simulink model "TST_CoME_ShutOff"  (R2016b)
settings: Solver=FixedStepDiscrete  StartTime=0.0  StopTime=simTime  FixedStep=sampleTime  RelTol=1e-3
values from neighbouring files (symbols this model uses):
  testCase = 1    [initTST_CoME_ShutOff_001.m]    (also in initTST_CoME_ShutOff_002.m = 2; initTST_CoME_ShutOff_003.m = 3; initTST_CoME_ShutOff_004.m = 4)
libraries: simulink x17, UnitTest_Lib x12
settings Model: Creator=zhengjinyan  LastModifiedBy=zhengjinyan
settings DebuggingCC: SignalRangeChecking=error

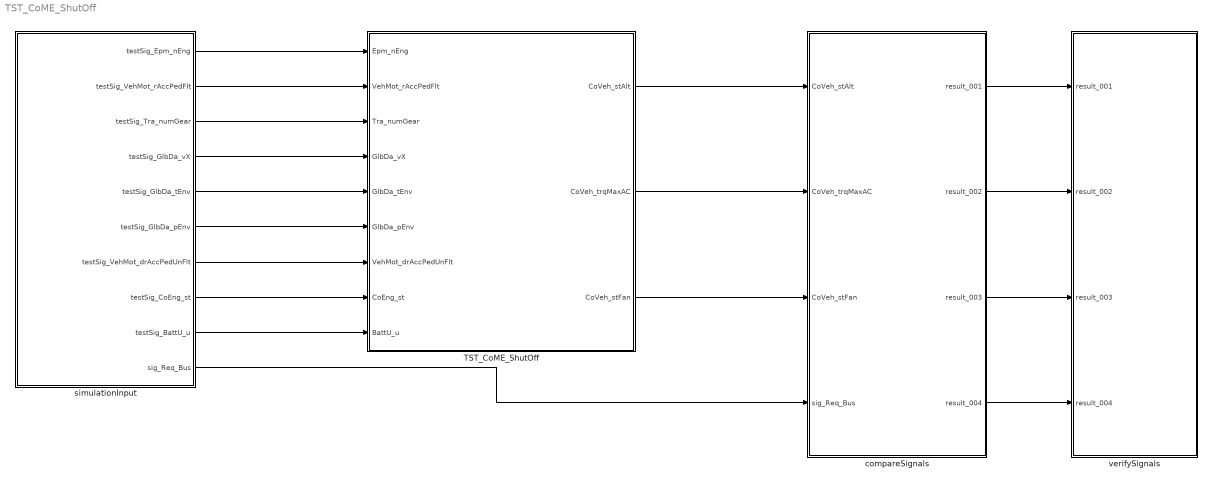
== system TST_CoME_ShutOff ==
  TST_CoME_ShutOff : Subsystem
  compareSignals : Subsystem
  simulationInput : Subsystem
  verifySignals : Subsystem
  wires:
  simulationInput/1(testSig_Epm_nEng) -> TST_CoME_ShutOff/1(Epm_nEng)
  simulationInput/2(testSig_VehMot_rAccPedFlt) -> TST_CoME_ShutOff/2(VehMot_rAccPedFlt)
  simulationInput/3(testSig_Tra_numGear) -> TST_CoME_ShutOff/3(Tra_numGear)
  simulationInput/4(testSig_GlbDa_vX) -> TST_CoME_ShutOff/4(GlbDa_vX)
  simulationInput/5(testSig_GlbDa_tEnv) -> TST_CoME_ShutOff/5(GlbDa_tEnv)
  simulationInput/6(testSig_GlbDa_pEnv) -> TST_CoME_ShutOff/6(GlbDa_pEnv)
  simulationInput/7(testSig_VehMot_drAccPedUnFlt) -> TST_CoME_ShutOff/7(VehMot_drAccPedUnFlt)
  simulationInput/8(testSig_CoEng_st) -> TST_CoME_ShutOff/8(CoEng_st)
  simulationInput/9(testSig_BattU_u) -> TST_CoME_ShutOff/9(BattU_u)
  TST_CoME_ShutOff/1(CoVeh_stAlt) -> compareSignals/1(CoVeh_stAlt)
  TST_CoME_ShutOff/2(CoVeh_trqMaxAC) -> compareSignals/2(CoVeh_trqMaxAC)
  TST_CoME_ShutOff/3(CoVeh_stFan) -> compareSignals/3(CoVeh_stFan)
  simulationInput/10(sig_Req_Bus) -> compareSignals/4(sig_Req_Bus)
  compareSignals/1(result_001) -> verifySignals/1(result_001)
  compareSignals/2(result_002) -> verifySignals/2(result_002)
  compareSignals/3(result_003) -> verifySignals/3(result_003)
  compareSignals/4(result_004) -> verifySignals/4(result_004)

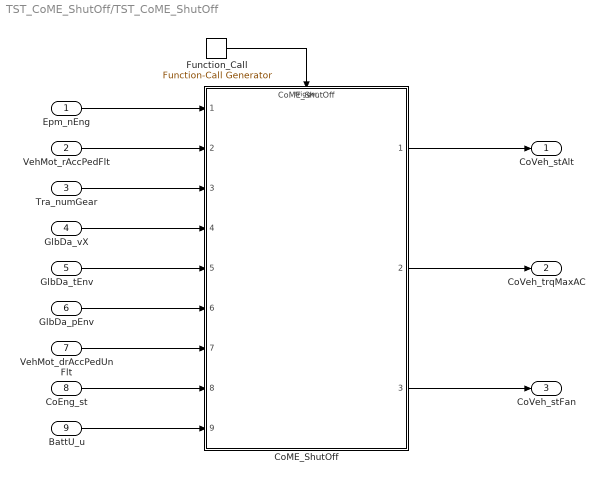
== system TST_CoME_ShutOff/TST_CoME_ShutOff ==
  Epm_nEng : Inport
  VehMot_rAccPedFlt : Inport  Port=2
  Tra_numGear : Inport  Port=3
  GlbDa_vX : Inport  Port=4
  GlbDa_tEnv : Inport  Port=5
  GlbDa_pEnv : Inport  Port=6
  VehMot_drAccPedUnFlt : Inport  Port=7
  CoEng_st : Inport  Port=8
  BattU_u : Inport  Port=9
  CoME_ShutOff : ModelReference  ModelNameDialog=CoME_ShutOff  SimulationMode=Normal  ModelReferenceVersion=1.29  TriggerPortName=function  TriggerPortTriggerType=function-call  TriggerPortStatesWhenEnabling=held
  Function_Call : simulink/Ports & Subsystems/Function-Call Generator  sample_time=sampleTime  numberOfIterations=1
  CoVeh_stAlt : Outport
  CoVeh_trqMaxAC : Outport  Port=2
  CoVeh_stFan : Outport  Port=3
  wires:
  Function_Call/1 -> CoME_ShutOff/Trigger
  Epm_nEng/1 -> CoME_ShutOff/1
  VehMot_rAccPedFlt/1 -> CoME_ShutOff/2
  Tra_numGear/1 -> CoME_ShutOff/3
  GlbDa_vX/1 -> CoME_ShutOff/4
  GlbDa_tEnv/1 -> CoME_ShutOff/5
  GlbDa_pEnv/1 -> CoME_ShutOff/6
  VehMot_drAccPedUnFlt/1 -> CoME_ShutOff/7
  CoEng_st/1 -> CoME_ShutOff/8
  BattU_u/1 -> CoME_ShutOff/9
  CoME_ShutOff/1 -> CoVeh_stAlt/1
  CoME_ShutOff/2 -> CoVeh_trqMaxAC/1
  CoME_ShutOff/3 -> CoVeh_stFan/1

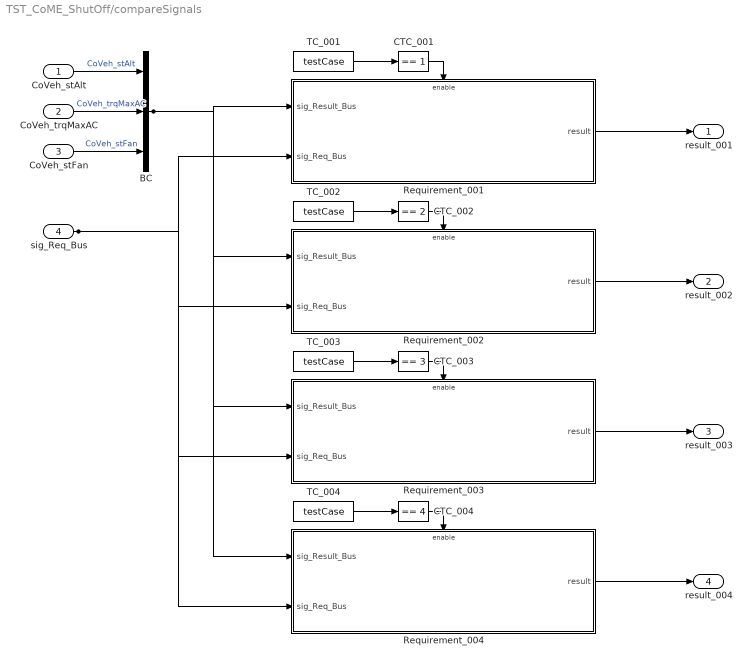
== system TST_CoME_ShutOff/compareSignals ==
  CoVeh_stAlt : Inport
  CoVeh_trqMaxAC : Inport  Port=2
  CoVeh_stFan : Inport  Port=3
  sig_Req_Bus : Inport  Port=4
  BC : BusCreator  Inputs=3
  CTC_001 : simulink/Logic and Bit Operations/Compare To Constant  relop===  const=1  OutDataTypeStr=boolean
  CTC_002 : simulink/Logic and Bit Operations/Compare To Constant  relop===  const=2  OutDataTypeStr=boolean
  CTC_003 : simulink/Logic and Bit Operations/Compare To Constant  relop===  const=3  OutDataTypeStr=boolean
  CTC_004 : simulink/Logic and Bit Operations/Compare To Constant  relop===  const=4  OutDataTypeStr=boolean
  Requirement_001 : Subsystem
  Requirement_002 : Subsystem
  Requirement_003 : Subsystem
  Requirement_004 : Subsystem
  TC_001 : Constant  Value=testCase
  TC_002 : Constant  Value=testCase
  TC_003 : Constant  Value=testCase
  TC_004 : Constant  Value=testCase
  result_001 : Outport
  result_002 : Outport  Port=2
  result_003 : Outport  Port=3
  result_004 : Outport  Port=4
  wires:
  CoVeh_stAlt/1 -> BC/1  "CoVeh_stAlt"
  CoVeh_trqMaxAC/1 -> BC/2  "CoVeh_trqMaxAC"
  CoVeh_stFan/1 -> BC/3  "CoVeh_stFan"
  TC_001/1 -> CTC_001/1
  CTC_001/1 -> Requirement_001/Enable
  sig_Req_Bus/1 -> Requirement_001/2(sig_Req_Bus), Requirement_002/2(sig_Req_Bus), Requirement_003/2(sig_Req_Bus), Requirement_004/2(sig_Req_Bus)
  BC/1 -> Requirement_001/1(sig_Result_Bus), Requirement_002/1(sig_Result_Bus), Requirement_003/1(sig_Result_Bus), Requirement_004/1(sig_Result_Bus)
  Requirement_001/1(result) -> result_001/1
  TC_002/1 -> CTC_002/1
  CTC_002/1 -> Requirement_002/Enable
  Requirement_002/1(result) -> result_002/1
  TC_003/1 -> CTC_003/1
  CTC_003/1 -> Requirement_003/Enable
  Requirement_003/1(result) -> result_003/1
  TC_004/1 -> CTC_004/1
  CTC_004/1 -> Requirement_004/Enable
  Requirement_004/1(result) -> result_004/1

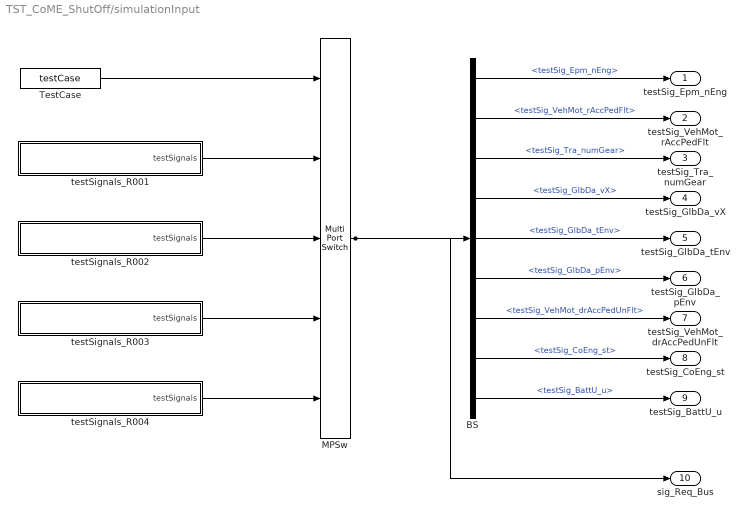
== system TST_CoME_ShutOff/simulationInput ==
  BS : BusSelector  OutputSignals=testSig_Epm_nEng,testSig_VehMot_rAccPedFlt,testSig_Tra_numGear,testSig_GlbDa_vX,testSig_GlbDa_tEnv,testSig_GlbDa_pEnv,testSig_VehMot_drAccPedUnFlt,testSig_CoEng_st,testSig_BattU_u
  MPSw : MultiPortSwitch  Inputs=4  SaturateOnIntegerOverflow=on  InputSameDT=on
  TestCase : Constant  Value=testCase
  testSignals_R001 : Subsystem
  testSignals_R002 : Subsystem
  testSignals_R003 : Subsystem
  testSignals_R004 : Subsystem
  testSig_Epm_nEng : Outport
  testSig_VehMot_rAccPedFlt : Outport  Port=2
  testSig_Tra_numGear : Outport  Port=3
  testSig_GlbDa_vX : Outport  Port=4
  testSig_GlbDa_tEnv : Outport  Port=5
  testSig_GlbDa_pEnv : Outport  Port=6
  testSig_VehMot_drAccPedUnFlt : Outport  Port=7
  testSig_CoEng_st : Outport  Port=8
  testSig_BattU_u : Outport  Port=9
  sig_Req_Bus : Outport  Port=10
  wires:
  BS/1 -> testSig_Epm_nEng/1  "<testSig_Epm_nEng>"
  BS/2 -> testSig_VehMot_rAccPedFlt/1  "<testSig_VehMot_rAccPedFlt>"
  BS/3 -> testSig_Tra_numGear/1  "<testSig_Tra_numGear>"
  BS/4 -> testSig_GlbDa_vX/1  "<testSig_GlbDa_vX>"
  BS/5 -> testSig_GlbDa_tEnv/1  "<testSig_GlbDa_tEnv>"
  BS/6 -> testSig_GlbDa_pEnv/1  "<testSig_GlbDa_pEnv>"
  BS/7 -> testSig_VehMot_drAccPedUnFlt/1  "<testSig_VehMot_drAccPedUnFlt>"
  BS/8 -> testSig_CoEng_st/1  "<testSig_CoEng_st>"
  BS/9 -> testSig_BattU_u/1  "<testSig_BattU_u>"
  MPSw/1 -> BS/1, sig_Req_Bus/1
  TestCase/1 -> MPSw/1
  testSignals_R001/1(testSignals) -> MPSw/2
  testSignals_R002/1(testSignals) -> MPSw/3
  testSignals_R003/1(testSignals) -> MPSw/4
  testSignals_R004/1(testSignals) -> MPSw/5

== system TST_CoME_ShutOff/verifySignals ==
  result_001 : Inport
  result_002 : Inport  Port=2
  result_003 : Inport  Port=3
  result_004 : Inport  Port=4
  Assertion_001 : Assertion  Enabled=off
  Assertion_002 : Assertion  Enabled=off
  Assertion_003 : Assertion  Enabled=off
  Assertion_004 : Assertion  Enabled=off
  wires:
  result_001/1 -> Assertion_001/1
  result_002/1 -> Assertion_002/1
  result_003/1 -> Assertion_003/1
  result_004/1 -> Assertion_004/1

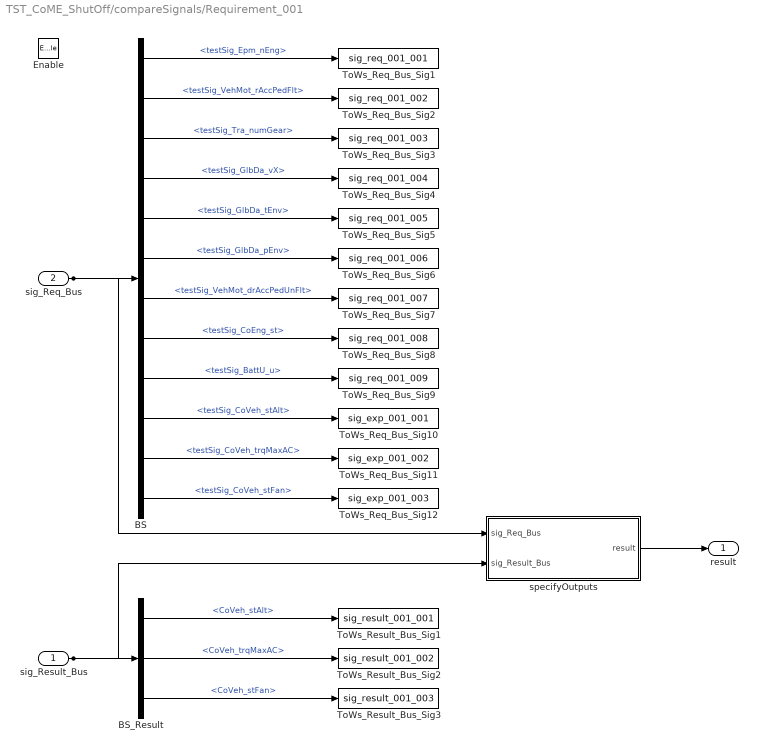
== system TST_CoME_ShutOff/compareSignals/Requirement_001 ==
  sig_Result_Bus : Inport
  sig_Req_Bus : Inport  Port=2
  Enable : EnablePort
  BS : BusSelector  OutputSignals=testSig_Epm_nEng,testSig_VehMot_rAccPedFlt,testSig_Tra_numGear,testSig_GlbDa_vX,testSig_GlbDa_tEnv,testSig_GlbDa_pEnv,testSig_VehMot_drAccPedUnFlt,testSig_CoEng_st,testSig_BattU_u,testSig_CoVeh_stAlt,testSig_CoVeh_trqMaxAC,testSig_CoVeh_stFan
  BS_Result : BusSelector  OutputSignals=CoVeh_stAlt,CoVeh_trqMaxAC,CoVeh_stFan
  ToWs_Req_Bus_Sig1 : ToWorkspace  VariableName=sig_req_001_001  SaveFormat=Structure With Time
  ToWs_Req_Bus_Sig10 : ToWorkspace  VariableName=sig_exp_001_001  SaveFormat=Structure With Time
  ToWs_Req_Bus_Sig11 : ToWorkspace  VariableName=sig_exp_001_002  SaveFormat=Structure With Time
  ToWs_Req_Bus_Sig12 : ToWorkspace  VariableName=sig_exp_001_003  SaveFormat=Structure With Time
  ToWs_Req_Bus_Sig2 : ToWorkspace  VariableName=sig_req_001_002  SaveFormat=Structure With Time
  ToWs_Req_Bus_Sig3 : ToWorkspace  VariableName=sig_req_001_003  SaveFormat=Structure With Time
  ToWs_Req_Bus_Sig4 : ToWorkspace  VariableName=sig_req_001_004  SaveFormat=Structure With Time
  ToWs_Req_Bus_Sig5 : ToWorkspace  VariableName=sig_req_001_005  SaveFormat=Structure With Time
  ToWs_Req_Bus_Sig6 : ToWorkspace  VariableName=sig_req_001_006  SaveFormat=Structure With Time
  ToWs_Req_Bus_Sig7 : ToWorkspace  VariableName=sig_req_001_007  SaveFormat=Structure With Time
  ToWs_Req_Bus_Sig8 : ToWorkspace  VariableName=sig_req_001_008  SaveFormat=Structure With Time
  ToWs_Req_Bus_Sig9 : ToWorkspace  VariableName=sig_req_001_009  SaveFormat=Structure With Time
  ToWs_Result_Bus_Sig1 : ToWorkspace  VariableName=sig_result_001_001  SaveFormat=Structure With Time
  ToWs_Result_Bus_Sig2 : ToWorkspace  VariableName=sig_result_001_002  SaveFormat=Structure With Time
  ToWs_Result_Bus_Sig3 : ToWorkspace  VariableName=sig_result_001_003  SaveFormat=Structure With Time
  specifyOutputs : Subsystem
  result : Outport
  wires:
  sig_Req_Bus/1 -> BS/1, specifyOutputs/1(sig_Req_Bus)
  BS/1 -> ToWs_Req_Bus_Sig1/1  "<testSig_Epm_nEng>"
  BS/2 -> ToWs_Req_Bus_Sig2/1  "<testSig_VehMot_rAccPedFlt>"
  BS/3 -> ToWs_Req_Bus_Sig3/1  "<testSig_Tra_numGear>"
  BS/4 -> ToWs_Req_Bus_Sig4/1  "<testSig_GlbDa_vX>"
  BS/5 -> ToWs_Req_Bus_Sig5/1  "<testSig_GlbDa_tEnv>"
  BS/6 -> ToWs_Req_Bus_Sig6/1  "<testSig_GlbDa_pEnv>"
  BS/7 -> ToWs_Req_Bus_Sig7/1  "<testSig_VehMot_drAccPedUnFlt>"
  BS/8 -> ToWs_Req_Bus_Sig8/1  "<testSig_CoEng_st>"
  BS/9 -> ToWs_Req_Bus_Sig9/1  "<testSig_BattU_u>"
  BS/10 -> ToWs_Req_Bus_Sig10/1  "<testSig_CoVeh_stAlt>"
  BS/11 -> ToWs_Req_Bus_Sig11/1  "<testSig_CoVeh_trqMaxAC>"
  BS/12 -> ToWs_Req_Bus_Sig12/1  "<testSig_CoVeh_stFan>"
  sig_Result_Bus/1 -> BS_Result/1, specifyOutputs/2(sig_Result_Bus)
  BS_Result/1 -> ToWs_Result_Bus_Sig1/1  "<CoVeh_stAlt>"
  BS_Result/2 -> ToWs_Result_Bus_Sig2/1  "<CoVeh_trqMaxAC>"
  BS_Result/3 -> ToWs_Result_Bus_Sig3/1  "<CoVeh_stFan>"
  specifyOutputs/1(result) -> result/1

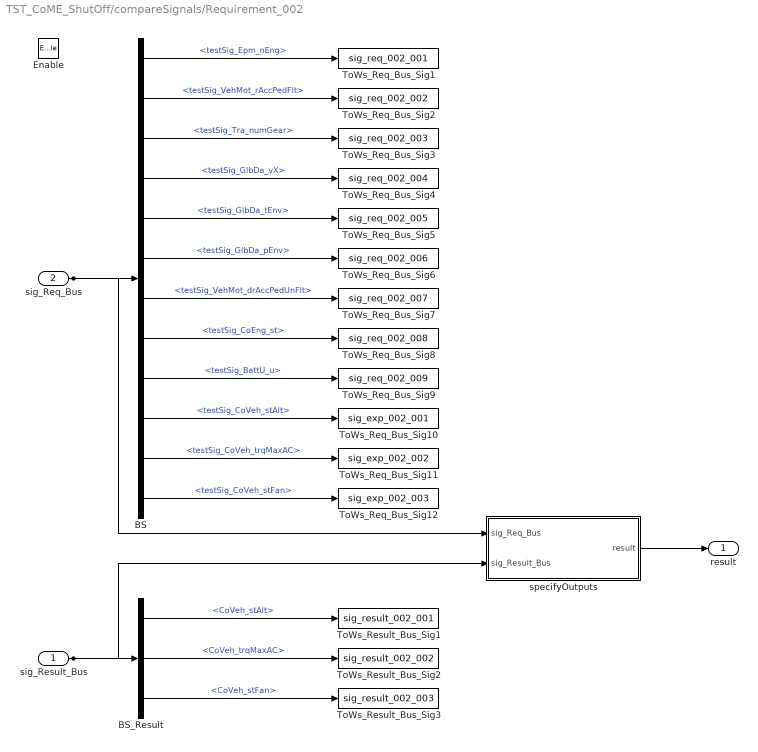
== system TST_CoME_ShutOff/compareSignals/Requirement_002 ==
  sig_Result_Bus : Inport
  sig_Req_Bus : Inport  Port=2
  Enable : EnablePort
  BS : BusSelector  OutputSignals=testSig_Epm_nEng,testSig_VehMot_rAccPedFlt,testSig_Tra_numGear,testSig_GlbDa_vX,testSig_GlbDa_tEnv,testSig_GlbDa_pEnv,testSig_VehMot_drAccPedUnFlt,testSig_CoEng_st,testSig_BattU_u,testSig_CoVeh_stAlt,testSig_CoVeh_trqMaxAC,testSig_CoVeh_stFan
  BS_Result : BusSelector  OutputSignals=CoVeh_stAlt,CoVeh_trqMaxAC,CoVeh_stFan
  ToWs_Req_Bus_Sig1 : ToWorkspace  VariableName=sig_req_002_001  SaveFormat=Structure With Time
  ToWs_Req_Bus_Sig10 : ToWorkspace  VariableName=sig_exp_002_001  SaveFormat=Structure With Time
  ToWs_Req_Bus_Sig11 : ToWorkspace  VariableName=sig_exp_002_002  SaveFormat=Structure With Time
  ToWs_Req_Bus_Sig12 : ToWorkspace  VariableName=sig_exp_002_003  SaveFormat=Structure With Time
  ToWs_Req_Bus_Sig2 : ToWorkspace  VariableName=sig_req_002_002  SaveFormat=Structure With Time
  ToWs_Req_Bus_Sig3 : ToWorkspace  VariableName=sig_req_002_003  SaveFormat=Structure With Time
  ToWs_Req_Bus_Sig4 : ToWorkspace  VariableName=sig_req_002_004  SaveFormat=Structure With Time
  ToWs_Req_Bus_Sig5 : ToWorkspace  VariableName=sig_req_002_005  SaveFormat=Structure With Time
  ToWs_Req_Bus_Sig6 : ToWorkspace  VariableName=sig_req_002_006  SaveFormat=Structure With Time
  ToWs_Req_Bus_Sig7 : ToWorkspace  VariableName=sig_req_002_007  SaveFormat=Structure With Time
  ToWs_Req_Bus_Sig8 : ToWorkspace  VariableName=sig_req_002_008  SaveFormat=Structure With Time
  ToWs_Req_Bus_Sig9 : ToWorkspace  VariableName=sig_req_002_009  SaveFormat=Structure With Time
  ToWs_Result_Bus_Sig1 : ToWorkspace  VariableName=sig_result_002_001  SaveFormat=Structure With Time
  ToWs_Result_Bus_Sig2 : ToWorkspace  VariableName=sig_result_002_002  SaveFormat=Structure With Time
  ToWs_Result_Bus_Sig3 : ToWorkspace  VariableName=sig_result_002_003  SaveFormat=Structure With Time
  specifyOutputs : Subsystem
  result : Outport
  wires:
  sig_Req_Bus/1 -> BS/1, specifyOutputs/1(sig_Req_Bus)
  BS/1 -> ToWs_Req_Bus_Sig1/1  "<testSig_Epm_nEng>"
  BS/2 -> ToWs_Req_Bus_Sig2/1  "<testSig_VehMot_rAccPedFlt>"
  BS/3 -> ToWs_Req_Bus_Sig3/1  "<testSig_Tra_numGear>"
  BS/4 -> ToWs_Req_Bus_Sig4/1  "<testSig_GlbDa_vX>"
  BS/5 -> ToWs_Req_Bus_Sig5/1  "<testSig_GlbDa_tEnv>"
  BS/6 -> ToWs_Req_Bus_Sig6/1  "<testSig_GlbDa_pEnv>"
  BS/7 -> ToWs_Req_Bus_Sig7/1  "<testSig_VehMot_drAccPedUnFlt>"
  BS/8 -> ToWs_Req_Bus_Sig8/1  "<testSig_CoEng_st>"
  BS/9 -> ToWs_Req_Bus_Sig9/1  "<testSig_BattU_u>"
  BS/10 -> ToWs_Req_Bus_Sig10/1  "<testSig_CoVeh_stAlt>"
  BS/11 -> ToWs_Req_Bus_Sig11/1  "<testSig_CoVeh_trqMaxAC>"
  BS/12 -> ToWs_Req_Bus_Sig12/1  "<testSig_CoVeh_stFan>"
  sig_Result_Bus/1 -> BS_Result/1, specifyOutputs/2(sig_Result_Bus)
  BS_Result/1 -> ToWs_Result_Bus_Sig1/1  "<CoVeh_stAlt>"
  BS_Result/2 -> ToWs_Result_Bus_Sig2/1  "<CoVeh_trqMaxAC>"
  BS_Result/3 -> ToWs_Result_Bus_Sig3/1  "<CoVeh_stFan>"
  specifyOutputs/1(result) -> result/1

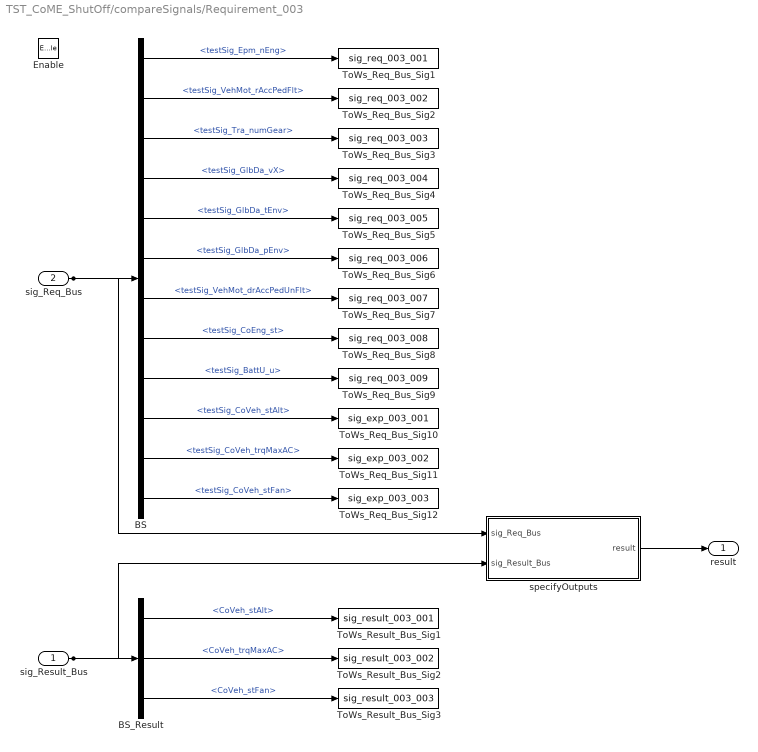
== system TST_CoME_ShutOff/compareSignals/Requirement_003 ==
  sig_Result_Bus : Inport
  sig_Req_Bus : Inport  Port=2
  Enable : EnablePort
  BS : BusSelector  OutputSignals=testSig_Epm_nEng,testSig_VehMot_rAccPedFlt,testSig_Tra_numGear,testSig_GlbDa_vX,testSig_GlbDa_tEnv,testSig_GlbDa_pEnv,testSig_VehMot_drAccPedUnFlt,testSig_CoEng_st,testSig_BattU_u,testSig_CoVeh_stAlt,testSig_CoVeh_trqMaxAC,testSig_CoVeh_stFan
  BS_Result : BusSelector  OutputSignals=CoVeh_stAlt,CoVeh_trqMaxAC,CoVeh_stFan
  ToWs_Req_Bus_Sig1 : ToWorkspace  VariableName=sig_req_003_001  SaveFormat=Structure With Time
  ToWs_Req_Bus_Sig10 : ToWorkspace  VariableName=sig_exp_003_001  SaveFormat=Structure With Time
  ToWs_Req_Bus_Sig11 : ToWorkspace  VariableName=sig_exp_003_002  SaveFormat=Structure With Time
  ToWs_Req_Bus_Sig12 : ToWorkspace  VariableName=sig_exp_003_003  SaveFormat=Structure With Time
  ToWs_Req_Bus_Sig2 : ToWorkspace  VariableName=sig_req_003_002  SaveFormat=Structure With Time
  ToWs_Req_Bus_Sig3 : ToWorkspace  VariableName=sig_req_003_003  SaveFormat=Structure With Time
  ToWs_Req_Bus_Sig4 : ToWorkspace  VariableName=sig_req_003_004  SaveFormat=Structure With Time
  ToWs_Req_Bus_Sig5 : ToWorkspace  VariableName=sig_req_003_005  SaveFormat=Structure With Time
  ToWs_Req_Bus_Sig6 : ToWorkspace  VariableName=sig_req_003_006  SaveFormat=Structure With Time
  ToWs_Req_Bus_Sig7 : ToWorkspace  VariableName=sig_req_003_007  SaveFormat=Structure With Time
  ToWs_Req_Bus_Sig8 : ToWorkspace  VariableName=sig_req_003_008  SaveFormat=Structure With Time
  ToWs_Req_Bus_Sig9 : ToWorkspace  VariableName=sig_req_003_009  SaveFormat=Structure With Time
  ToWs_Result_Bus_Sig1 : ToWorkspace  VariableName=sig_result_003_001  SaveFormat=Structure With Time
  ToWs_Result_Bus_Sig2 : ToWorkspace  VariableName=sig_result_003_002  SaveFormat=Structure With Time
  ToWs_Result_Bus_Sig3 : ToWorkspace  VariableName=sig_result_003_003  SaveFormat=Structure With Time
  specifyOutputs : Subsystem
  result : Outport
  wires:
  sig_Req_Bus/1 -> BS/1, specifyOutputs/1(sig_Req_Bus)
  BS/1 -> ToWs_Req_Bus_Sig1/1  "<testSig_Epm_nEng>"
  BS/2 -> ToWs_Req_Bus_Sig2/1  "<testSig_VehMot_rAccPedFlt>"
  BS/3 -> ToWs_Req_Bus_Sig3/1  "<testSig_Tra_numGear>"
  BS/4 -> ToWs_Req_Bus_Sig4/1  "<testSig_GlbDa_vX>"
  BS/5 -> ToWs_Req_Bus_Sig5/1  "<testSig_GlbDa_tEnv>"
  BS/6 -> ToWs_Req_Bus_Sig6/1  "<testSig_GlbDa_pEnv>"
  BS/7 -> ToWs_Req_Bus_Sig7/1  "<testSig_VehMot_drAccPedUnFlt>"
  BS/8 -> ToWs_Req_Bus_Sig8/1  "<testSig_CoEng_st>"
  BS/9 -> ToWs_Req_Bus_Sig9/1  "<testSig_BattU_u>"
  BS/10 -> ToWs_Req_Bus_Sig10/1  "<testSig_CoVeh_stAlt>"
  BS/11 -> ToWs_Req_Bus_Sig11/1  "<testSig_CoVeh_trqMaxAC>"
  BS/12 -> ToWs_Req_Bus_Sig12/1  "<testSig_CoVeh_stFan>"
  sig_Result_Bus/1 -> BS_Result/1, specifyOutputs/2(sig_Result_Bus)
  BS_Result/1 -> ToWs_Result_Bus_Sig1/1  "<CoVeh_stAlt>"
  BS_Result/2 -> ToWs_Result_Bus_Sig2/1  "<CoVeh_trqMaxAC>"
  BS_Result/3 -> ToWs_Result_Bus_Sig3/1  "<CoVeh_stFan>"
  specifyOutputs/1(result) -> result/1

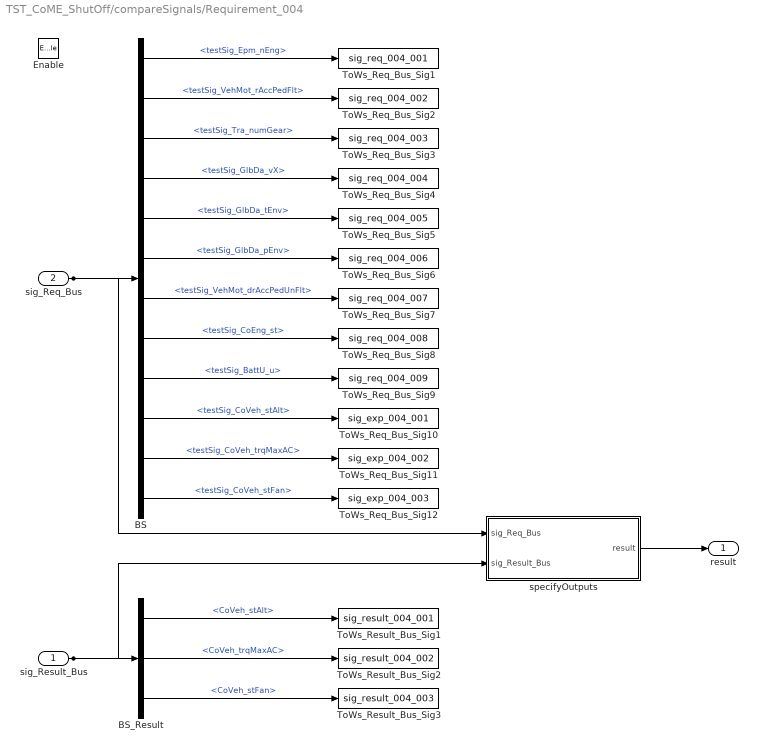
== system TST_CoME_ShutOff/compareSignals/Requirement_004 ==
  sig_Result_Bus : Inport
  sig_Req_Bus : Inport  Port=2
  Enable : EnablePort
  BS : BusSelector  OutputSignals=testSig_Epm_nEng,testSig_VehMot_rAccPedFlt,testSig_Tra_numGear,testSig_GlbDa_vX,testSig_GlbDa_tEnv,testSig_GlbDa_pEnv,testSig_VehMot_drAccPedUnFlt,testSig_CoEng_st,testSig_BattU_u,testSig_CoVeh_stAlt,testSig_CoVeh_trqMaxAC,testSig_CoVeh_stFan
  BS_Result : BusSelector  OutputSignals=CoVeh_stAlt,CoVeh_trqMaxAC,CoVeh_stFan
  ToWs_Req_Bus_Sig1 : ToWorkspace  VariableName=sig_req_004_001  SaveFormat=Structure With Time
  ToWs_Req_Bus_Sig10 : ToWorkspace  VariableName=sig_exp_004_001  SaveFormat=Structure With Time
  ToWs_Req_Bus_Sig11 : ToWorkspace  VariableName=sig_exp_004_002  SaveFormat=Structure With Time
  ToWs_Req_Bus_Sig12 : ToWorkspace  VariableName=sig_exp_004_003  SaveFormat=Structure With Time
  ToWs_Req_Bus_Sig2 : ToWorkspace  VariableName=sig_req_004_002  SaveFormat=Structure With Time
  ToWs_Req_Bus_Sig3 : ToWorkspace  VariableName=sig_req_004_003  SaveFormat=Structure With Time
  ToWs_Req_Bus_Sig4 : ToWorkspace  VariableName=sig_req_004_004  SaveFormat=Structure With Time
  ToWs_Req_Bus_Sig5 : ToWorkspace  VariableName=sig_req_004_005  SaveFormat=Structure With Time
  ToWs_Req_Bus_Sig6 : ToWorkspace  VariableName=sig_req_004_006  SaveFormat=Structure With Time
  ToWs_Req_Bus_Sig7 : ToWorkspace  VariableName=sig_req_004_007  SaveFormat=Structure With Time
  ToWs_Req_Bus_Sig8 : ToWorkspace  VariableName=sig_req_004_008  SaveFormat=Structure With Time
  ToWs_Req_Bus_Sig9 : ToWorkspace  VariableName=sig_req_004_009  SaveFormat=Structure With Time
  ToWs_Result_Bus_Sig1 : ToWorkspace  VariableName=sig_result_004_001  SaveFormat=Structure With Time
  ToWs_Result_Bus_Sig2 : ToWorkspace  VariableName=sig_result_004_002  SaveFormat=Structure With Time
  ToWs_Result_Bus_Sig3 : ToWorkspace  VariableName=sig_result_004_003  SaveFormat=Structure With Time
  specifyOutputs : Subsystem
  result : Outport
  wires:
  sig_Req_Bus/1 -> BS/1, specifyOutputs/1(sig_Req_Bus)
  BS/1 -> ToWs_Req_Bus_Sig1/1  "<testSig_Epm_nEng>"
  BS/2 -> ToWs_Req_Bus_Sig2/1  "<testSig_VehMot_rAccPedFlt>"
  BS/3 -> ToWs_Req_Bus_Sig3/1  "<testSig_Tra_numGear>"
  BS/4 -> ToWs_Req_Bus_Sig4/1  "<testSig_GlbDa_vX>"
  BS/5 -> ToWs_Req_Bus_Sig5/1  "<testSig_GlbDa_tEnv>"
  BS/6 -> ToWs_Req_Bus_Sig6/1  "<testSig_GlbDa_pEnv>"
  BS/7 -> ToWs_Req_Bus_Sig7/1  "<testSig_VehMot_drAccPedUnFlt>"
  BS/8 -> ToWs_Req_Bus_Sig8/1  "<testSig_CoEng_st>"
  BS/9 -> ToWs_Req_Bus_Sig9/1  "<testSig_BattU_u>"
  BS/10 -> ToWs_Req_Bus_Sig10/1  "<testSig_CoVeh_stAlt>"
  BS/11 -> ToWs_Req_Bus_Sig11/1  "<testSig_CoVeh_trqMaxAC>"
  BS/12 -> ToWs_Req_Bus_Sig12/1  "<testSig_CoVeh_stFan>"
  sig_Result_Bus/1 -> BS_Result/1, specifyOutputs/2(sig_Result_Bus)
  BS_Result/1 -> ToWs_Result_Bus_Sig1/1  "<CoVeh_stAlt>"
  BS_Result/2 -> ToWs_Result_Bus_Sig2/1  "<CoVeh_trqMaxAC>"
  BS_Result/3 -> ToWs_Result_Bus_Sig3/1  "<CoVeh_stFan>"
  specifyOutputs/1(result) -> result/1

== system TST_CoME_ShutOff/simulationInput/testSignals_R001 ==
  BC : BusCreator  Inputs=12
  spec_BattU_u : FromWorkspace  VariableName=testSig_BattU_u  Interpolate=off  OutputAfterFinalValue=Holding final value
  spec_CoEng_st : FromWorkspace  VariableName=testSig_CoEng_st  Interpolate=off  OutputAfterFinalValue=Holding final value
  spec_CoVeh_stAlt : FromWorkspace  VariableName=testSig_CoVeh_stAlt  Interpolate=off  OutputAfterFinalValue=Holding final value
  spec_CoVeh_stFan : FromWorkspace  VariableName=testSig_CoVeh_stFan  Interpolate=off  OutputAfterFinalValue=Holding final value
  spec_CoVeh_trqMaxAC : FromWorkspace  VariableName=testSig_CoVeh_trqMaxAC  Interpolate=off  OutputAfterFinalValue=Holding final value
  spec_Epm_nEng : FromWorkspace  VariableName=testSig_Epm_nEng  Interpolate=off  OutputAfterFinalValue=Holding final value
  spec_GlbDa_pEnv : FromWorkspace  VariableName=testSig_GlbDa_pEnv  Interpolate=off  OutputAfterFinalValue=Holding final value
  spec_GlbDa_tEnv : FromWorkspace  VariableName=testSig_GlbDa_tEnv  Interpolate=off  OutputAfterFinalValue=Holding final value
  spec_GlbDa_vX : FromWorkspace  VariableName=testSig_GlbDa_vX  Interpolate=off  OutputAfterFinalValue=Holding final value
  spec_Tra_numGear : FromWorkspace  VariableName=testSig_Tra_numGear  Interpolate=off  OutputAfterFinalValue=Holding final value
  spec_VehMot_drAccPedUnFlt : FromWorkspace  VariableName=testSig_VehMot_drAccPedUnFlt  Interpolate=off  OutputAfterFinalValue=Holding final value
  spec_VehMot_rAccPedFlt : FromWorkspace  VariableName=testSig_VehMot_rAccPedFlt  Interpolate=off  OutputAfterFinalValue=Holding final value
  testSignals : Outport
  wires:
  BC/1 -> testSignals/1
  spec_Epm_nEng/1 -> BC/1  "testSig_Epm_nEng"
  spec_VehMot_rAccPedFlt/1 -> BC/2  "testSig_VehMot_rAccPedFlt"
  spec_Tra_numGear/1 -> BC/3  "testSig_Tra_numGear"
  spec_GlbDa_vX/1 -> BC/4  "testSig_GlbDa_vX"
  spec_GlbDa_tEnv/1 -> BC/5  "testSig_GlbDa_tEnv"
  spec_GlbDa_pEnv/1 -> BC/6  "testSig_GlbDa_pEnv"
  spec_VehMot_drAccPedUnFlt/1 -> BC/7  "testSig_VehMot_drAccPedUnFlt"
  spec_CoEng_st/1 -> BC/8  "testSig_CoEng_st"
  spec_BattU_u/1 -> BC/9  "testSig_BattU_u"
  spec_CoVeh_stAlt/1 -> BC/10  "testSig_CoVeh_stAlt"
  spec_CoVeh_trqMaxAC/1 -> BC/11  "testSig_CoVeh_trqMaxAC"
  spec_CoVeh_stFan/1 -> BC/12  "testSig_CoVeh_stFan"

== system TST_CoME_ShutOff/simulationInput/testSignals_R002 ==
  BC : BusCreator  Inputs=12
  spec_BattU_u : FromWorkspace  VariableName=testSig_BattU_u  Interpolate=off  OutputAfterFinalValue=Holding final value
  spec_CoEng_st : FromWorkspace  VariableName=testSig_CoEng_st  Interpolate=off  OutputAfterFinalValue=Holding final value
  spec_CoVeh_stAlt : FromWorkspace  VariableName=testSig_CoVeh_stAlt  Interpolate=off  OutputAfterFinalValue=Holding final value
  spec_CoVeh_stFan : FromWorkspace  VariableName=testSig_CoVeh_stFan  Interpolate=off  OutputAfterFinalValue=Holding final value
  spec_CoVeh_trqMaxAC : FromWorkspace  VariableName=testSig_CoVeh_trqMaxAC  Interpolate=off  OutputAfterFinalValue=Holding final value
  spec_Epm_nEng : FromWorkspace  VariableName=testSig_Epm_nEng  Interpolate=off  OutputAfterFinalValue=Holding final value
  spec_GlbDa_pEnv : FromWorkspace  VariableName=testSig_GlbDa_pEnv  Interpolate=off  OutputAfterFinalValue=Holding final value
  spec_GlbDa_tEnv : FromWorkspace  VariableName=testSig_GlbDa_tEnv  Interpolate=off  OutputAfterFinalValue=Holding final value
  spec_GlbDa_vX : FromWorkspace  VariableName=testSig_GlbDa_vX  Interpolate=off  OutputAfterFinalValue=Holding final value
  spec_Tra_numGear : FromWorkspace  VariableName=testSig_Tra_numGear  Interpolate=off  OutputAfterFinalValue=Holding final value
  spec_VehMot_drAccPedUnFlt : FromWorkspace  VariableName=testSig_VehMot_drAccPedUnFlt  Interpolate=off  OutputAfterFinalValue=Holding final value
  spec_VehMot_rAccPedFlt : FromWorkspace  VariableName=testSig_VehMot_rAccPedFlt  Interpolate=off  OutputAfterFinalValue=Holding final value
  testSignals : Outport
  wires:
  BC/1 -> testSignals/1
  spec_Epm_nEng/1 -> BC/1  "testSig_Epm_nEng"
  spec_VehMot_rAccPedFlt/1 -> BC/2  "testSig_VehMot_rAccPedFlt"
  spec_Tra_numGear/1 -> BC/3  "testSig_Tra_numGear"
  spec_GlbDa_vX/1 -> BC/4  "testSig_GlbDa_vX"
  spec_GlbDa_tEnv/1 -> BC/5  "testSig_GlbDa_tEnv"
  spec_GlbDa_pEnv/1 -> BC/6  "testSig_GlbDa_pEnv"
  spec_VehMot_drAccPedUnFlt/1 -> BC/7  "testSig_VehMot_drAccPedUnFlt"
  spec_CoEng_st/1 -> BC/8  "testSig_CoEng_st"
  spec_BattU_u/1 -> BC/9  "testSig_BattU_u"
  spec_CoVeh_stAlt/1 -> BC/10  "testSig_CoVeh_stAlt"
  spec_CoVeh_trqMaxAC/1 -> BC/11  "testSig_CoVeh_trqMaxAC"
  spec_CoVeh_stFan/1 -> BC/12  "testSig_CoVeh_stFan"

== system TST_CoME_ShutOff/simulationInput/testSignals_R003 ==
  BC : BusCreator  Inputs=12
  spec_BattU_u : FromWorkspace  VariableName=testSig_BattU_u  Interpolate=off  OutputAfterFinalValue=Holding final value
  spec_CoEng_st : FromWorkspace  VariableName=testSig_CoEng_st  Interpolate=off  OutputAfterFinalValue=Holding final value
  spec_CoVeh_stAlt : FromWorkspace  VariableName=testSig_CoVeh_stAlt  Interpolate=off  OutputAfterFinalValue=Holding final value
  spec_CoVeh_stFan : FromWorkspace  VariableName=testSig_CoVeh_stFan  Interpolate=off  OutputAfterFinalValue=Holding final value
  spec_CoVeh_trqMaxAC : FromWorkspace  VariableName=testSig_CoVeh_trqMaxAC  Interpolate=off  OutputAfterFinalValue=Holding final value
  spec_Epm_nEng : FromWorkspace  VariableName=testSig_Epm_nEng  Interpolate=off  OutputAfterFinalValue=Holding final value
  spec_GlbDa_pEnv : FromWorkspace  VariableName=testSig_GlbDa_pEnv  Interpolate=off  OutputAfterFinalValue=Holding final value
  spec_GlbDa_tEnv : FromWorkspace  VariableName=testSig_GlbDa_tEnv  Interpolate=off  OutputAfterFinalValue=Holding final value
  spec_GlbDa_vX : FromWorkspace  VariableName=testSig_GlbDa_vX  Interpolate=off  OutputAfterFinalValue=Holding final value
  spec_Tra_numGear : FromWorkspace  VariableName=testSig_Tra_numGear  Interpolate=off  OutputAfterFinalValue=Holding final value
  spec_VehMot_drAccPedUnFlt : FromWorkspace  VariableName=testSig_VehMot_drAccPedUnFlt  Interpolate=off  OutputAfterFinalValue=Holding final value
  spec_VehMot_rAccPedFlt : FromWorkspace  VariableName=testSig_VehMot_rAccPedFlt  Interpolate=off  OutputAfterFinalValue=Holding final value
  testSignals : Outport
  wires:
  BC/1 -> testSignals/1
  spec_Epm_nEng/1 -> BC/1  "testSig_Epm_nEng"
  spec_VehMot_rAccPedFlt/1 -> BC/2  "testSig_VehMot_rAccPedFlt"
  spec_Tra_numGear/1 -> BC/3  "testSig_Tra_numGear"
  spec_GlbDa_vX/1 -> BC/4  "testSig_GlbDa_vX"
  spec_GlbDa_tEnv/1 -> BC/5  "testSig_GlbDa_tEnv"
  spec_GlbDa_pEnv/1 -> BC/6  "testSig_GlbDa_pEnv"
  spec_VehMot_drAccPedUnFlt/1 -> BC/7  "testSig_VehMot_drAccPedUnFlt"
  spec_CoEng_st/1 -> BC/8  "testSig_CoEng_st"
  spec_BattU_u/1 -> BC/9  "testSig_BattU_u"
  spec_CoVeh_stAlt/1 -> BC/10  "testSig_CoVeh_stAlt"
  spec_CoVeh_trqMaxAC/1 -> BC/11  "testSig_CoVeh_trqMaxAC"
  spec_CoVeh_stFan/1 -> BC/12  "testSig_CoVeh_stFan"

== system TST_CoME_ShutOff/simulationInput/testSignals_R004 ==
  BC : BusCreator  Inputs=12
  spec_BattU_u : FromWorkspace  VariableName=testSig_BattU_u  Interpolate=off  OutputAfterFinalValue=Holding final value
  spec_CoEng_st : FromWorkspace  VariableName=testSig_CoEng_st  Interpolate=off  OutputAfterFinalValue=Holding final value
  spec_CoVeh_stAlt : FromWorkspace  VariableName=testSig_CoVeh_stAlt  Interpolate=off  OutputAfterFinalValue=Holding final value
  spec_CoVeh_stFan : FromWorkspace  VariableName=testSig_CoVeh_stFan  Interpolate=off  OutputAfterFinalValue=Holding final value
  spec_CoVeh_trqMaxAC : FromWorkspace  VariableName=testSig_CoVeh_trqMaxAC  Interpolate=off  OutputAfterFinalValue=Holding final value
  spec_Epm_nEng : FromWorkspace  VariableName=testSig_Epm_nEng  Interpolate=off  OutputAfterFinalValue=Holding final value
  spec_GlbDa_pEnv : FromWorkspace  VariableName=testSig_GlbDa_pEnv  Interpolate=off  OutputAfterFinalValue=Holding final value
  spec_GlbDa_tEnv : FromWorkspace  VariableName=testSig_GlbDa_tEnv  Interpolate=off  OutputAfterFinalValue=Holding final value
  spec_GlbDa_vX : FromWorkspace  VariableName=testSig_GlbDa_vX  Interpolate=off  OutputAfterFinalValue=Holding final value
  spec_Tra_numGear : FromWorkspace  VariableName=testSig_Tra_numGear  Interpolate=off  OutputAfterFinalValue=Holding final value
  spec_VehMot_drAccPedUnFlt : FromWorkspace  VariableName=testSig_VehMot_drAccPedUnFlt  Interpolate=off  OutputAfterFinalValue=Holding final value
  spec_VehMot_rAccPedFlt : FromWorkspace  VariableName=testSig_VehMot_rAccPedFlt  Interpolate=off  OutputAfterFinalValue=Holding final value
  testSignals : Outport
  wires:
  BC/1 -> testSignals/1
  spec_Epm_nEng/1 -> BC/1  "testSig_Epm_nEng"
  spec_VehMot_rAccPedFlt/1 -> BC/2  "testSig_VehMot_rAccPedFlt"
  spec_Tra_numGear/1 -> BC/3  "testSig_Tra_numGear"
  spec_GlbDa_vX/1 -> BC/4  "testSig_GlbDa_vX"
  spec_GlbDa_tEnv/1 -> BC/5  "testSig_GlbDa_tEnv"
  spec_GlbDa_pEnv/1 -> BC/6  "testSig_GlbDa_pEnv"
  spec_VehMot_drAccPedUnFlt/1 -> BC/7  "testSig_VehMot_drAccPedUnFlt"
  spec_CoEng_st/1 -> BC/8  "testSig_CoEng_st"
  spec_BattU_u/1 -> BC/9  "testSig_BattU_u"
  spec_CoVeh_stAlt/1 -> BC/10  "testSig_CoVeh_stAlt"
  spec_CoVeh_trqMaxAC/1 -> BC/11  "testSig_CoVeh_trqMaxAC"
  spec_CoVeh_stFan/1 -> BC/12  "testSig_CoVeh_stFan"

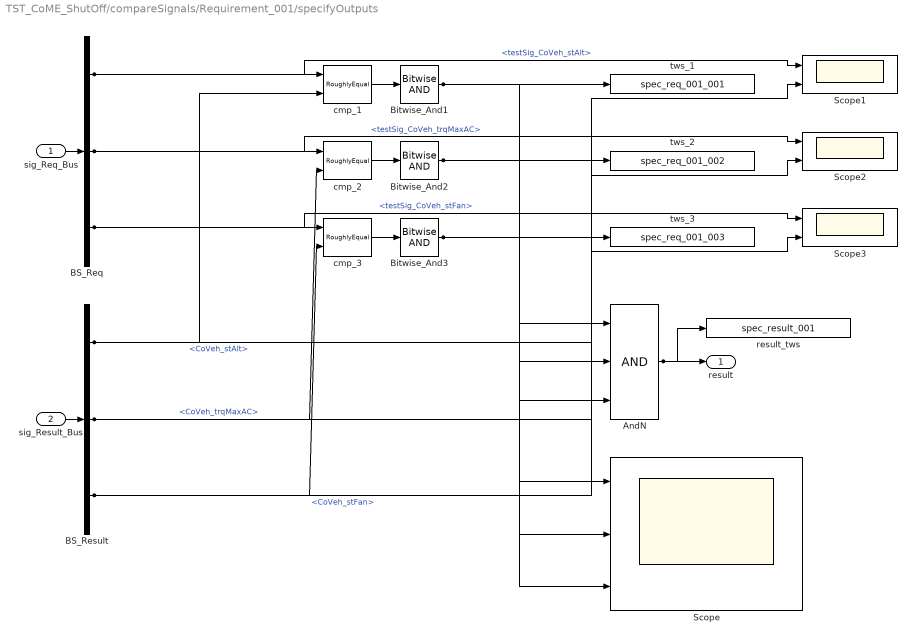
== system TST_CoME_ShutOff/compareSignals/Requirement_001/specifyOutputs ==
  sig_Req_Bus : Inport
  sig_Result_Bus : Inport  Port=2
  AndN : Logic  Inputs=3
  BS_Req : BusSelector  OutputSignals=testSig_CoVeh_stAlt,testSig_CoVeh_trqMaxAC,testSig_CoVeh_stFan
  BS_Result : BusSelector  OutputSignals=CoVeh_stAlt,CoVeh_trqMaxAC,CoVeh_stFan
  Bitwise_And1 : simulink/Logic and Bit Operations/Bitwise Operator  logicop=AND  UseBitMask=off  BitMask=bin2dec('11011001')  BitMaskRealWorld=Stored Integer
  Bitwise_And2 : simulink/Logic and Bit Operations/Bitwise Operator  logicop=AND  UseBitMask=off  BitMask=bin2dec('11011001')  BitMaskRealWorld=Stored Integer
  Bitwise_And3 : simulink/Logic and Bit Operations/Bitwise Operator  logicop=AND  UseBitMask=off  BitMask=bin2dec('11011001')  BitMaskRealWorld=Stored Integer
  Scope : Scope  NumInputPorts=3
  Scope1 : Scope  NumInputPorts=2
  Scope2 : Scope  NumInputPorts=2
  Scope3 : Scope  NumInputPorts=2
  cmp_1 : UnitTest_Lib/RoughlyEqual  slope=0.1
  cmp_2 : UnitTest_Lib/RoughlyEqual  slope=0.1
  cmp_3 : UnitTest_Lib/RoughlyEqual  slope=0.1
  result_tws : ToWorkspace  VariableName=spec_result_001
  tws_1 : ToWorkspace  VariableName=spec_req_001_001
  tws_2 : ToWorkspace  VariableName=spec_req_001_002
  tws_3 : ToWorkspace  VariableName=spec_req_001_003
  result : Outport
  wires:
  sig_Req_Bus/1 -> BS_Req/1
  sig_Result_Bus/1 -> BS_Result/1
  AndN/1 -> result/1, result_tws/1
  BS_Req/1 -> cmp_1/1, Scope1/1  "<testSig_CoVeh_stAlt>"
  BS_Result/1 -> cmp_1/2, Scope1/2  "<CoVeh_stAlt>"
  cmp_1/1 -> Bitwise_And1/1
  Bitwise_And1/1 -> tws_1/1, AndN/1, Scope/1
  BS_Req/2 -> cmp_2/1, Scope2/1  "<testSig_CoVeh_trqMaxAC>"
  BS_Result/2 -> cmp_2/2, Scope2/2  "<CoVeh_trqMaxAC>"
  cmp_2/1 -> Bitwise_And2/1
  Bitwise_And2/1 -> tws_2/1, AndN/2, Scope/2
  BS_Req/3 -> cmp_3/1, Scope3/1  "<testSig_CoVeh_stFan>"
  BS_Result/3 -> cmp_3/2, Scope3/2  "<CoVeh_stFan>"
  cmp_3/1 -> Bitwise_And3/1
  Bitwise_And3/1 -> tws_3/1, AndN/3, Scope/3

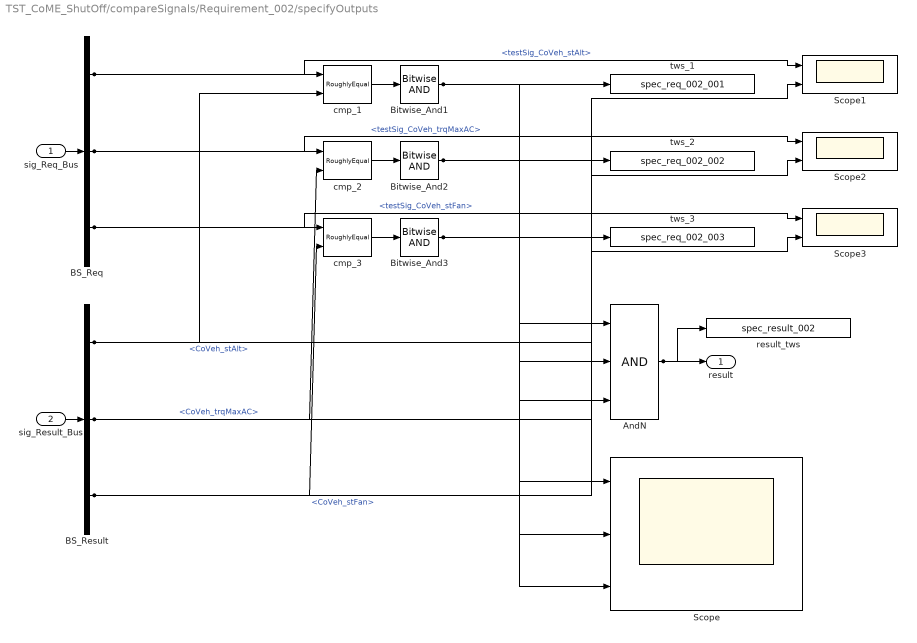
== system TST_CoME_ShutOff/compareSignals/Requirement_002/specifyOutputs ==
  sig_Req_Bus : Inport
  sig_Result_Bus : Inport  Port=2
  AndN : Logic  Inputs=3
  BS_Req : BusSelector  OutputSignals=testSig_CoVeh_stAlt,testSig_CoVeh_trqMaxAC,testSig_CoVeh_stFan
  BS_Result : BusSelector  OutputSignals=CoVeh_stAlt,CoVeh_trqMaxAC,CoVeh_stFan
  Bitwise_And1 : simulink/Logic and Bit Operations/Bitwise Operator  logicop=AND  UseBitMask=off  BitMask=bin2dec('11011001')  BitMaskRealWorld=Stored Integer
  Bitwise_And2 : simulink/Logic and Bit Operations/Bitwise Operator  logicop=AND  UseBitMask=off  BitMask=bin2dec('11011001')  BitMaskRealWorld=Stored Integer
  Bitwise_And3 : simulink/Logic and Bit Operations/Bitwise Operator  logicop=AND  UseBitMask=off  BitMask=bin2dec('11011001')  BitMaskRealWorld=Stored Integer
  Scope : Scope  NumInputPorts=3
  Scope1 : Scope  NumInputPorts=2
  Scope2 : Scope  NumInputPorts=2
  Scope3 : Scope  NumInputPorts=2
  cmp_1 : UnitTest_Lib/RoughlyEqual  slope=0.1
  cmp_2 : UnitTest_Lib/RoughlyEqual  slope=0.1
  cmp_3 : UnitTest_Lib/RoughlyEqual  slope=0.1
  result_tws : ToWorkspace  VariableName=spec_result_002
  tws_1 : ToWorkspace  VariableName=spec_req_002_001
  tws_2 : ToWorkspace  VariableName=spec_req_002_002
  tws_3 : ToWorkspace  VariableName=spec_req_002_003
  result : Outport
  wires:
  sig_Req_Bus/1 -> BS_Req/1
  sig_Result_Bus/1 -> BS_Result/1
  AndN/1 -> result/1, result_tws/1
  BS_Req/1 -> cmp_1/1, Scope1/1  "<testSig_CoVeh_stAlt>"
  BS_Result/1 -> cmp_1/2, Scope1/2  "<CoVeh_stAlt>"
  cmp_1/1 -> Bitwise_And1/1
  Bitwise_And1/1 -> tws_1/1, AndN/1, Scope/1
  BS_Req/2 -> cmp_2/1, Scope2/1  "<testSig_CoVeh_trqMaxAC>"
  BS_Result/2 -> cmp_2/2, Scope2/2  "<CoVeh_trqMaxAC>"
  cmp_2/1 -> Bitwise_And2/1
  Bitwise_And2/1 -> tws_2/1, AndN/2, Scope/2
  BS_Req/3 -> cmp_3/1, Scope3/1  "<testSig_CoVeh_stFan>"
  BS_Result/3 -> cmp_3/2, Scope3/2  "<CoVeh_stFan>"
  cmp_3/1 -> Bitwise_And3/1
  Bitwise_And3/1 -> tws_3/1, AndN/3, Scope/3

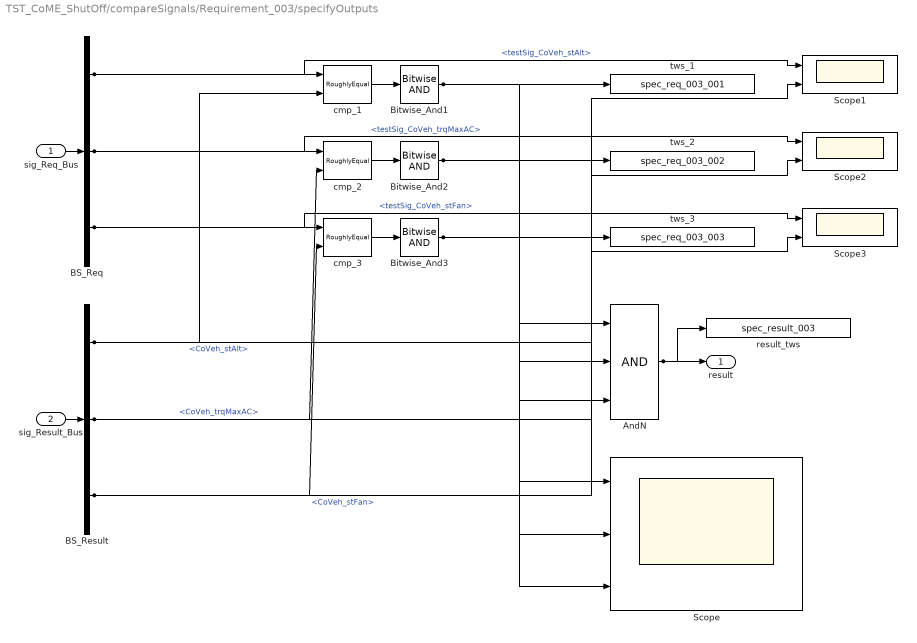
== system TST_CoME_ShutOff/compareSignals/Requirement_003/specifyOutputs ==
  sig_Req_Bus : Inport
  sig_Result_Bus : Inport  Port=2
  AndN : Logic  Inputs=3
  BS_Req : BusSelector  OutputSignals=testSig_CoVeh_stAlt,testSig_CoVeh_trqMaxAC,testSig_CoVeh_stFan
  BS_Result : BusSelector  OutputSignals=CoVeh_stAlt,CoVeh_trqMaxAC,CoVeh_stFan
  Bitwise_And1 : simulink/Logic and Bit Operations/Bitwise Operator  logicop=AND  UseBitMask=off  BitMask=bin2dec('11011001')  BitMaskRealWorld=Stored Integer
  Bitwise_And2 : simulink/Logic and Bit Operations/Bitwise Operator  logicop=AND  UseBitMask=off  BitMask=bin2dec('11011001')  BitMaskRealWorld=Stored Integer
  Bitwise_And3 : simulink/Logic and Bit Operations/Bitwise Operator  logicop=AND  UseBitMask=off  BitMask=bin2dec('11011001')  BitMaskRealWorld=Stored Integer
  Scope : Scope  NumInputPorts=3
  Scope1 : Scope  NumInputPorts=2
  Scope2 : Scope  NumInputPorts=2
  Scope3 : Scope  NumInputPorts=2
  cmp_1 : UnitTest_Lib/RoughlyEqual  slope=0.1
  cmp_2 : UnitTest_Lib/RoughlyEqual  slope=0.1
  cmp_3 : UnitTest_Lib/RoughlyEqual  slope=0.1
  result_tws : ToWorkspace  VariableName=spec_result_003
  tws_1 : ToWorkspace  VariableName=spec_req_003_001
  tws_2 : ToWorkspace  VariableName=spec_req_003_002
  tws_3 : ToWorkspace  VariableName=spec_req_003_003
  result : Outport
  wires:
  sig_Req_Bus/1 -> BS_Req/1
  sig_Result_Bus/1 -> BS_Result/1
  AndN/1 -> result/1, result_tws/1
  BS_Req/1 -> cmp_1/1, Scope1/1  "<testSig_CoVeh_stAlt>"
  BS_Result/1 -> cmp_1/2, Scope1/2  "<CoVeh_stAlt>"
  cmp_1/1 -> Bitwise_And1/1
  Bitwise_And1/1 -> tws_1/1, AndN/1, Scope/1
  BS_Req/2 -> cmp_2/1, Scope2/1  "<testSig_CoVeh_trqMaxAC>"
  BS_Result/2 -> cmp_2/2, Scope2/2  "<CoVeh_trqMaxAC>"
  cmp_2/1 -> Bitwise_And2/1
  Bitwise_And2/1 -> tws_2/1, AndN/2, Scope/2
  BS_Req/3 -> cmp_3/1, Scope3/1  "<testSig_CoVeh_stFan>"
  BS_Result/3 -> cmp_3/2, Scope3/2  "<CoVeh_stFan>"
  cmp_3/1 -> Bitwise_And3/1
  Bitwise_And3/1 -> tws_3/1, AndN/3, Scope/3

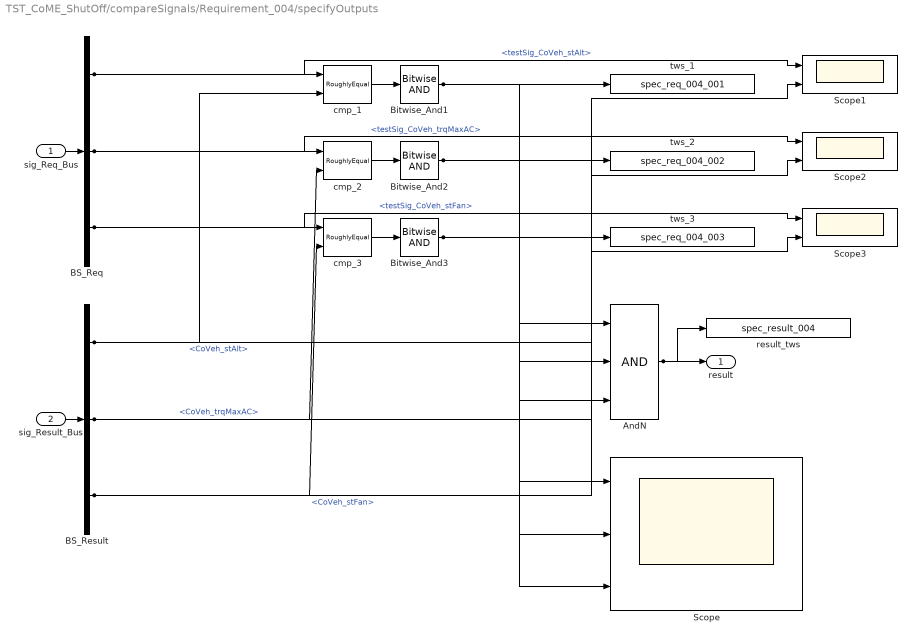
== system TST_CoME_ShutOff/compareSignals/Requirement_004/specifyOutputs ==
  sig_Req_Bus : Inport
  sig_Result_Bus : Inport  Port=2
  AndN : Logic  Inputs=3
  BS_Req : BusSelector  OutputSignals=testSig_CoVeh_stAlt,testSig_CoVeh_trqMaxAC,testSig_CoVeh_stFan
  BS_Result : BusSelector  OutputSignals=CoVeh_stAlt,CoVeh_trqMaxAC,CoVeh_stFan
  Bitwise_And1 : simulink/Logic and Bit Operations/Bitwise Operator  logicop=AND  UseBitMask=off  BitMask=bin2dec('11011001')  BitMaskRealWorld=Stored Integer
  Bitwise_And2 : simulink/Logic and Bit Operations/Bitwise Operator  logicop=AND  UseBitMask=off  BitMask=bin2dec('11011001')  BitMaskRealWorld=Stored Integer
  Bitwise_And3 : simulink/Logic and Bit Operations/Bitwise Operator  logicop=AND  UseBitMask=off  BitMask=bin2dec('11011001')  BitMaskRealWorld=Stored Integer
  Scope : Scope  NumInputPorts=3
  Scope1 : Scope  NumInputPorts=2
  Scope2 : Scope  NumInputPorts=2
  Scope3 : Scope  NumInputPorts=2
  cmp_1 : UnitTest_Lib/RoughlyEqual  slope=0.1
  cmp_2 : UnitTest_Lib/RoughlyEqual  slope=0.1
  cmp_3 : UnitTest_Lib/RoughlyEqual  slope=0.1
  result_tws : ToWorkspace  VariableName=spec_result_004
  tws_1 : ToWorkspace  VariableName=spec_req_004_001
  tws_2 : ToWorkspace  VariableName=spec_req_004_002
  tws_3 : ToWorkspace  VariableName=spec_req_004_003
  result : Outport
  wires:
  sig_Req_Bus/1 -> BS_Req/1
  sig_Result_Bus/1 -> BS_Result/1
  AndN/1 -> result/1, result_tws/1
  BS_Req/1 -> cmp_1/1, Scope1/1  "<testSig_CoVeh_stAlt>"
  BS_Result/1 -> cmp_1/2, Scope1/2  "<CoVeh_stAlt>"
  cmp_1/1 -> Bitwise_And1/1
  Bitwise_And1/1 -> tws_1/1, AndN/1, Scope/1
  BS_Req/2 -> cmp_2/1, Scope2/1  "<testSig_CoVeh_trqMaxAC>"
  BS_Result/2 -> cmp_2/2, Scope2/2  "<CoVeh_trqMaxAC>"
  cmp_2/1 -> Bitwise_And2/1
  Bitwise_And2/1 -> tws_2/1, AndN/2, Scope/2
  BS_Req/3 -> cmp_3/1, Scope3/1  "<testSig_CoVeh_stFan>"
  BS_Result/3 -> cmp_3/2, Scope3/2  "<CoVeh_stFan>"
  cmp_3/1 -> Bitwise_And3/1
  Bitwise_And3/1 -> tws_3/1, AndN/3, Scope/3
